simulink model "funcion_5"  (R2019a)
settings: Solver=VariableStepAuto  StartTime=0.0  StopTime=1  RelTol=1e-3
values from neighbouring files (symbols this model uses):
  a = -2.0000e-01    (= -0.2)    [programa_nodos.m]
  h = 1.0000e+00    (= 1)    [programa_nodos.m]
  hdis = hdis'    [programa_nodos.m]
  i = 1.0000e+00    (= 1)    [programa_nodos.m]
  j = 1.0000e+00    (= 1)    [programa_nodos.m]
  o = 1.0000e+00    (= 1)    [programa_nodos.m]
  s = 1.3156e+02    (= 131.56)    [programa_nodos.m]
  tm = 0.5    [programa_nodos.m]
  v = 1.2563e+00    (= 1.2563)    [programa_nodos.m]
  z0 = 0.5    [programa_nodos.m]
  z1 = 0.00000001    (= 1e-08)    [programa_nodos.m]
  z2 = 0.00000001    (= 1e-08)    [programa_nodos.m]
  z3 = 0.00000001    (= 1e-08)    [programa_nodos.m]
  z4 = 0.00000001    (= 1e-08)    [programa_nodos.m]
  z5 = 0.00000001    (= 1e-08)    [programa_nodos.m]
  z6 = 0.00000001    (= 1e-08)    [programa_nodos.m]
  z7 = 0.00000001    (= 1e-08)    [programa_nodos.m]
undefined symbols (not defined in the file or in its folder): A, A2, adis, B, B2, bdis, C, C2, cdis, g
libraries: simulink x1
settings Model: Creator=Alejoxbg  LastModifiedBy=Alejoxbg

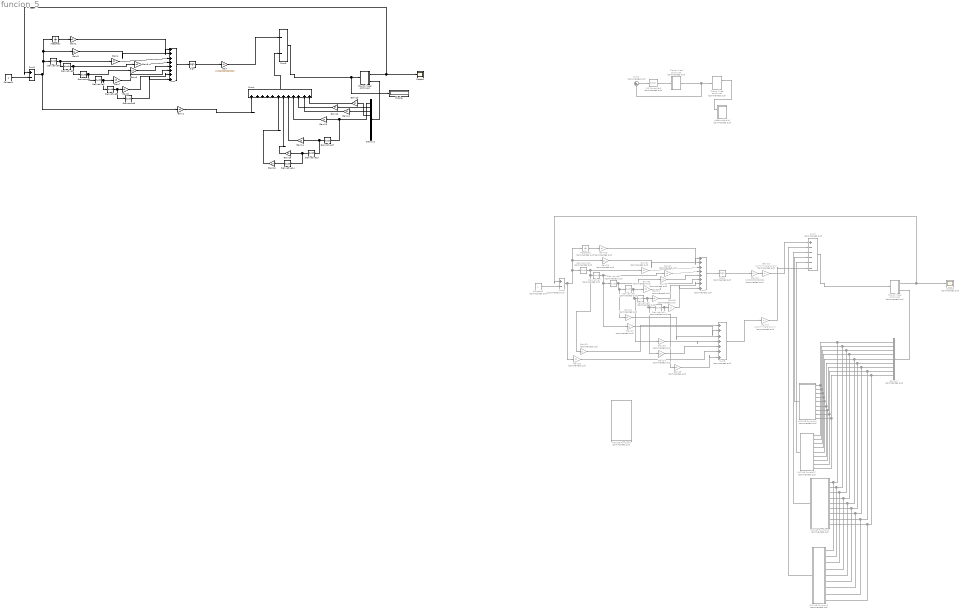
== system funcion_5 ==
  Constant : Constant
  Constant1 : Constant  Commented=on
  Demux1 : Demux  Commented=on  Outputs=9
  Demux2 : Demux  Outputs=9
  Derivative{1..6,13..14,17} (9 alike) : Derivative
  Derivative{7..12} (6 alike) : Derivative  Commented=on
  Display : Display
  Gain : Gain  Gain=0.0000000000001
  Gain1 : Gain  Gain=z0
  Gain10 : Gain  Gain=z1
  Gain11 : Gain  Gain=z2
  Gain12 : Gain  Gain=z3
  Gain13 : Gain  Gain=z4
  Gain14 : Gain  Gain=z5
  Gain15 : Gain  Gain=z6
  Gain16 : Gain  Gain=z7
  Gain18 : Gain  Commented=on  Gain=0.0000000000001
  Gain19 : Gain  Commented=on  Gain=1/(s*j*i*h*g*a*g*o*v)
  Gain2 : Gain  Gain=z0
  Gain20 : Gain  Commented=on  Gain=z1
  Gain21 : Gain  Commented=on  Gain=z2
  Gain22 : Gain  Commented=on  Gain=z3
  Gain23 : Gain  Commented=on  Gain=z4
  Gain24 : Gain  Commented=on  Gain=z5
  Gain25 : Gain  Commented=on  Gain=z6
  Gain26 : Gain  Commented=on  Gain=z0
  Gain27 : Gain  Commented=on  Gain=1/(s*j*i*h*g*a*g*o*v)
  Gain28 : Gain  Commented=on  Gain=z0
  Gain29 : Gain  Commented=on  Gain=z1
  Gain3 : Gain  Gain=z1
  Gain30 : Gain  Commented=on  Gain=z2
  Gain31 : Gain  Commented=on  Gain=z3
  Gain32 : Gain  Commented=on  Gain=z4
  Gain33 : Gain  Commented=on  Gain=z5
  Gain34 : Gain  Commented=on  Gain=z6
  Gain35 : Gain  Commented=on  Gain=z7
  Gain4 : Gain  Gain=z2
  Gain5 : Gain  Gain=z3
  Gain6 : Gain  Gain=z4
  Gain7 : Gain  Gain=z5
  Gain8 : Gain  Gain=z6
  Integrator : Integrator
  Integrator1 : Integrator  Commented=on
  MATLAB Function5 : MATLAB Function  Commented=on  TreatAsAtomicUnit=on
  MATLAB Function6 : MATLAB Function  Commented=on  TreatAsAtomicUnit=on
  MATLAB Function7 : MATLAB Function  Commented=on  TreatAsAtomicUnit=on
  MATLAB Function8 : MATLAB Function  Commented=on  TreatAsAtomicUnit=on
  MATLAB Function9 : MATLAB Function  Commented=on  TreatAsAtomicUnit=on
  PID Controller2 : simulink/Continuous/PID Controller  Commented=on  Controller=PID  Form=Parallel  TimeDomain=Continuous-time  SampleTime=-1  IntegratorMethod=Forward Euler  FilterMethod=Forward Euler  ControllerParametersSource=internal  P=12.1148539818802  I=1.25631014904339  D=27.6845650272969  UseFilter=on  N=4.3146205312046  TunerSelectOption=Transfer Function Based (PID Tuner App)  InitialConditionSource=internal  InitialConditionForIntegrator=0  InitialConditionForFilter=0  DifferentiatorICPrevScaledInput=0  ExternalReset=none  TrackingMode=off  Kt=1  LimitOutput=off  UpperSaturationLimit=inf  LowerSaturationLimit=-inf  LinearizeAsGain=on  AntiWindupMode=none  Kb=1  POutMin=[]  POutMax=[]  IOutMin=[]  IOutMax=[]  DOutMin=[]  DOutMax=[]  NOutMin=[]  NOutMax=[]  SumOutMin=[]  SumOutMax=[]  SaturationOutMin=[]  SaturationOutMax=[]  PParamMin=[]  PParamMax=[]  IParamMin=[]  IParamMax=[]  DParamMin=[]  DParamMax=[]  NParamMin=[]  NParamMax=[]  KbParamMin=[]  KbParamMax=[]  KtParamMin=[]  KtParamMax=[]  KbOutMin=[]  KbOutMax=[]  KtOutMin=[]  KtOutMax=[]  IntegratorOutMin=[]  IntegratorOutMax=[]  FilterOutMin=[]  FilterOutMax=[]  SumI1OutMin=[]  SumI1OutMax=[]  SumI2OutMin=[]  SumI2OutMax=[]  SumI3OutMin=[]  SumI3OutMax=[]  SumI4OutMin=[]  SumI4OutMax=[]  SumDOutMin=[]  SumDOutMax=[]  DifferentiatorOutMin=[]  DifferentiatorOutMax=[]  FilterDiffOutCoefMin=[]  FilterDiffOutCoefMax=[]  ReciprocalOutMin=[]  ReciprocalOutMax=[]  SumDenOutMin=[]  SumDenOutMax=[]  SumNumOutMin=[]  SumNumOutMax=[]  DivideOutMin=[]  DivideOutMax=[]  IntegratorContinuousStateAttributes=''  IntegratorStateMustResolveToSignalObject=off  IntegratorRTWStateStorageClass=Auto  FilterContinuousStateAttributes=''  FilterStateMustResolveToSignalObject=off  FilterRTWStateStorageClass=Auto  ParallelPVariant=InternalParameters  IdealPVariant=Disabled  IVariant=InternalParameters  DVariant=InternalParameters  IntegratorVariant=Continuous  SatVariant=Disabled  AWVariant=Passthrough  PCopyVariant=Disabled  TRVariant=Disabled  FdbkBlocksVariant=Forward  IdealPFdbkVariant=Disabled  SatFdbkVariant=Disabled  DerivativeFilterVariant=ContFilter  NVariant=InternalParameters  NCopyVariant=Disabled  FilterICVariant=InternalICsFilter  IntegratorICVariant=InternalICs  ExternalResetVariant=Disabled  TRSumVariant=Passthrough  SumFdbkVariant=Disabled  SumVariant=Sum_PID
  Planta lineal continua1 : Subsystem
  Planta lineal continua2 : Subsystem  Commented=on
  Planta lineal continua3 : Subsystem  Commented=on
  Planta lineal continua4 : Subsystem  Commented=on
  Scope1 : Scope
  Scope2 : Scope  Commented=on
  Sign : Signum  ZeroCross=off
  Sign1 : Signum  Commented=on  ZeroCross=off
  Sum : Sum  Inputs=|++++++++
  Sum1 : Sum  Commented=on  Inputs=|+-
  Sum2 : Sum  Inputs=|+-
  Sum3 : Sum  Inputs=|--
  Sum4 : Sum  Inputs=|++++++++++++
  Sum5 : Sum  Commented=on  Inputs=|++++++++
  Sum6 : Sum  Commented=on  Inputs=|+-
  Sum7 : Sum  Commented=on  Inputs=|+-----
  Sum8 : Sum  Commented=on  Inputs=|+++++++
  observadordis1 : Subsystem  Commented=on
  wires:
  Constant/1 -> Sum2/2
  Sum2/1 -> Gain1/1, Derivative6/1, Gain3/1, Integrator/1
  Integrator/1 -> Gain2/1
  Sum/1 -> Sign/1
  Sign/1 -> Gain/1
  Gain2/1 -> Sum/1
  Gain3/1 -> Sum/2
  Gain4/1 -> Sum/3
  Derivative6/1 -> Derivative1/1, Gain4/1
  Gain5/1 -> Sum/4
  Derivative1/1 -> Derivative4/1, Gain5/1
  Derivative4/1 -> Derivative2/1, Gain6/1
  Gain6/1 -> Sum/5
  Derivative2/1 -> Derivative3/1, Gain7/1
  Gain7/1 -> Sum/6
  Derivative3/1 -> Derivative5/1, Gain8/1
  Gain8/1 -> Sum/7
  Derivative5/1 -> Sum/8
  Gain/1 -> Sum3/1
  Sum3/1 -> Display/1, Planta lineal continua1/1(u)
  Sum1/1 -> PID Controller2/1
  Planta lineal continua3/1(y) -> Planta lineal continua4/1(u), Sum1/2
  ? -> Sum1/1
  PID Controller2/1 -> Planta lineal continua3/1(u)
  Planta lineal continua1/1(y) -> Sum2/1, Scope1/1
  Sum4/1 -> Sum3/2
  Gain23/1 -> Sum8/4
  Gain27/1 -> Sum7/6
  Demux1/8 -> MATLAB Function9/8(u8), MATLAB Function8/8(u8), MATLAB Function7/8(u8), MATLAB Function6/8(u8)
  Demux1/9 -> MATLAB Function9/9(u9), MATLAB Function8/9(u9), MATLAB Function7/9(u9), MATLAB Function6/9(u9)
  Gain33/1 -> Sum5/6
  Demux1/6 -> MATLAB Function9/6(u6), MATLAB Function8/6(u6), MATLAB Function7/6(u6), MATLAB Function6/6(u6)
  MATLAB Function6/1(y) -> Sum7/4
  MATLAB Function9/1(y) -> Sum7/2
  Demux1/2 -> MATLAB Function9/2(u2), MATLAB Function8/2(u2), MATLAB Function7/2(u2), MATLAB Function6/2(u2)
  Demux1/3 -> MATLAB Function9/3(u3), MATLAB Function8/3(u3), MATLAB Function7/3(u3), MATLAB Function6/3(u3)
  Gain29/1 -> Sum5/2
  Gain35/1 -> Sum5/8
  Sign1/1 -> Gain18/1
  Gain28/1 -> Sum5/1
  Gain34/1 -> Sum5/7
  Gain31/1 -> Sum5/4
  Constant1/1 -> Sum6/2
  Gain24/1 -> Sum8/5
  Derivative9/1 -> Gain24/1, Derivative11/1, Gain34/1
  Derivative10/1 -> Gain22/1, Derivative8/1, Gain32/1
  Demux1/4 -> MATLAB Function9/4(u4), MATLAB Function8/4(u4), MATLAB Function7/4(u4), MATLAB Function6/4(u4)
  Sum6/1 -> Gain26/1, Derivative12/1, Gain29/1, Integrator1/1
  Gain32/1 -> Sum5/5
  Planta lineal continua2/2(X) -> Demux1/1
  Gain25/1 -> Sum8/7
  Derivative8/1 -> Gain23/1, Derivative9/1, Gain33/1
  Planta lineal continua2/1(y) -> Sum6/1, Scope2/1
  Gain20/1 -> Sum8/1
  Gain21/1 -> Sum8/2
  Sum8/1 -> Gain27/1
  Demux1/5 -> MATLAB Function9/5(u5), MATLAB Function8/5(u5), MATLAB Function7/5(u5), MATLAB Function6/5(u5)
  Demux1/1 -> MATLAB Function9/1(u1), MATLAB Function8/1(u1), MATLAB Function7/1(u1), MATLAB Function6/1(u1)
  Demux1/7 -> MATLAB Function9/7(u7), MATLAB Function8/7(u7), MATLAB Function7/7(u7), MATLAB Function6/7(u7)
  Sum7/1 -> Planta lineal continua2/1(u)
  Derivative11/1 -> Gain25/1, Gain35/1
  Gain26/1 -> Sum8/6
  Gain30/1 -> Sum5/3
  Gain18/1 -> Gain19/1
  MATLAB Function7/1(y) -> Sum7/5
  Gain22/1 -> Sum8/3
  Derivative7/1 -> Gain21/1, Derivative10/1, Gain31/1
  MATLAB Function8/1(y) -> Sum7/3
  Gain19/1 -> Sum7/1
  Integrator1/1 -> Gain28/1
  Sum5/1 -> Sign1/1
  Derivative12/1 -> Gain20/1, Derivative7/1, Gain30/1
  Gain1/1 -> Sum4/1
  Planta lineal continua1/2(X) -> Demux2/1
  Demux2/4 -> Gain10/1
  Gain10/1 -> Sum4/12
  Demux2/3 -> Gain11/1
  Gain11/1 -> Sum4/11
  Demux2/2 -> Gain12/1
  Gain12/1 -> Sum4/10
  Gain13/1 -> Sum4/9
  Derivative17/1 -> Derivative13/1, Gain14/1
  Gain14/1 -> Sum4/8
  Gain15/1 -> Sum4/7
  Derivative14/1 -> Gain16/1
  Derivative13/1 -> Derivative14/1, Gain15/1
  Gain16/1 -> Sum4/6
  Planta lineal continua4/1(y) -> observadordis1/1(Y)
  ? -> observadordis1/2(U)
  Demux2/1 -> Derivative17/1, Gain13/1

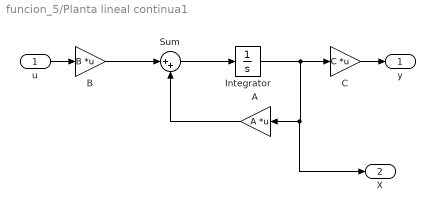
== system funcion_5/Planta lineal continua1 ==
  u : Inport
  A : Gain  Gain=A  Multiplication=Matrix(K*u) (u vector)
  B : Gain  Gain=B  Multiplication=Matrix(K*u) (u vector)
  C : Gain  Gain=C  Multiplication=Matrix(K*u) (u vector)
  Integrator : Integrator  InitialCondition=0.000001
  Sum : Sum  Inputs=|++
  y : Outport
  X : Outport  Port=2
  wires:
  C/1 -> y/1
  u/1 -> B/1
  Integrator/1 -> X/1, A/1, C/1
  A/1 -> Sum/2
  Sum/1 -> Integrator/1
  B/1 -> Sum/1

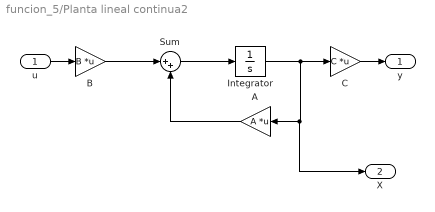
== system funcion_5/Planta lineal continua2 ==
  u : Inport
  A : Gain  Gain=A  Multiplication=Matrix(K*u) (u vector)
  B : Gain  Gain=B  Multiplication=Matrix(K*u) (u vector)
  C : Gain  Gain=C  Multiplication=Matrix(K*u) (u vector)
  Integrator : Integrator
  Sum : Sum  Inputs=|++
  y : Outport
  X : Outport  Port=2
  wires:
  C/1 -> y/1
  u/1 -> B/1
  Integrator/1 -> X/1, A/1, C/1
  A/1 -> Sum/2
  Sum/1 -> Integrator/1
  B/1 -> Sum/1

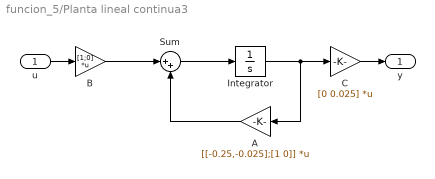
== system funcion_5/Planta lineal continua3 ==
  u : Inport
  A : Gain  Gain=[[-0.25,-0.025];[1 0]]  Multiplication=Matrix(K*u) (u vector)
  B : Gain  Gain=[1;0]  Multiplication=Matrix(K*u) (u vector)
  C : Gain  Gain=[0 0.025]  Multiplication=Matrix(K*u) (u vector)
  Integrator : Integrator
  Sum : Sum  Inputs=|++
  y : Outport
  wires:
  C/1 -> y/1
  u/1 -> B/1
  Integrator/1 -> A/1, C/1
  A/1 -> Sum/2
  Sum/1 -> Integrator/1
  B/1 -> Sum/1

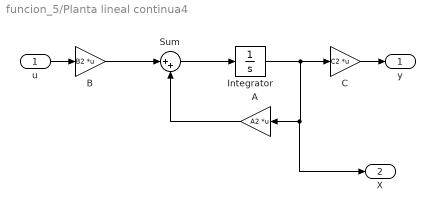
== system funcion_5/Planta lineal continua4 ==
  u : Inport
  A : Gain  Gain=A2  Multiplication=Matrix(K*u) (u vector)
  B : Gain  Gain=B2  Multiplication=Matrix(K*u) (u vector)
  C : Gain  Gain=C2  Multiplication=Matrix(K*u) (u vector)
  Integrator : Integrator
  Sum : Sum  Inputs=|++
  y : Outport
  X : Outport  Port=2
  wires:
  C/1 -> y/1
  u/1 -> B/1
  Integrator/1 -> X/1, A/1, C/1
  A/1 -> Sum/2
  Sum/1 -> Integrator/1
  B/1 -> Sum/1

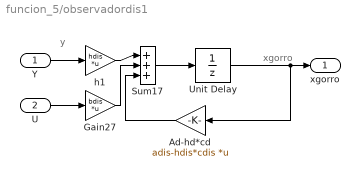
== system funcion_5/observadordis1 ==
  note: xgorro
  note: y
  Y : Inport
  U : Inport  Port=2
  Ad-hd*cd : Gain  Gain=adis-hdis*cdis  Multiplication=Matrix(K*u) (u vector)  SampleTime=tm
  Gain27 : Gain  Gain=bdis  Multiplication=Matrix(K*u) (u vector)  SampleTime=tm
  Sum17 : Sum  Inputs=|+++
  Unit Delay : UnitDelay  SampleTime=tm  HasFrameUpgradeWarning=on
  h1 : Gain  Gain=hdis  Multiplication=Matrix(K*u) (u vector)  SampleTime=tm
  xgorro : Outport
  wires:
  Sum17/1 -> Unit Delay/1
  h1/1 -> Sum17/1
  Unit Delay/1 -> Ad-hd*cd/1, xgorro/1
  Ad-hd*cd/1 -> Sum17/3
  Gain27/1 -> Sum17/2
  Y/1 -> h1/1
  U/1 -> Gain27/1

== matlab function funcion_5/MATLAB Function5 ==
  data: u1 input; y output; u2 input; u3 input; u4 input; u5 input; u6 input; u7 input; u8 input; u9 input
function y = fcn(u1,u2,u3,u4,u5,u6,u7,u8,u9)
  a=1.1520e-07
 b=-2.0000e-01
 c=-1.6000e-02  
 d=-6.4000e-04  
 e=-1.2800e-05  
 f=-1.0240e-07 
 g=2.5000e-02
 h=1.0000e+00
 i=1.0000e+00
 j=1.0000e+00
 k=1.0000e+00
 l=-2.5000e-01
 m=-3.3141e+00
 n=-4.3146e+00
 o=1.0000e+00
 p=1.0000e+00
 q=-2.9862e+00
 r=-4.3146e+00
 s=-3.1408e-02
 t=1.3156e+02
 u=1.1945e+02
 v=1.2563e+00
y = s*j*i*h*g*a*a*(a*u1+b*u2+c*u3+d*u4+e*u5+g*u7)+s*j*i*h*g*a*(b*g*u1+c*h*u2+d*i*u3+e*j*u4+g*o*u6)+s*j*i*h*g*a*(d*h*g*u1+d*h*u2+d*i*u3)+s*j*i*h*g*a*g*o*(k*u6+l*u7+m*u8+n*u9)+s*j*i*h*g*a*g*o*v*u;

== matlab function funcion_5/MATLAB Function6 ==
  data: u1 input; y output; u2 input; u3 input; u4 input; u5 input; u6 input; u7 input; u8 input; u9 input
function y = fcn(u1,u2,u3,u4,u5,u6,u7,u8,u9)
a=1.1520e-07
 b=-2.0000e-01
 c=-1.6000e-02  
 d=-6.4000e-04  
 e=-1.2800e-05  
 f=-1.0240e-07 
 g=2.5000e-02
 h=1.0000e+00
 i=1.0000e+00
 j=1.0000e+00
 k=1.0000e+00
 l=-2.5000e-01
 m=-3.3141e+00
 n=-4.3146e+00
 o=1.0000e+00
 p=1.0000e+00
 q=-2.9862e+00
 r=-4.3146e+00
 s=-3.1408e-02
 t=1.3156e+02
 u=1.1945e+02
 v=1.2563e+00
y = a/(g*o*v)*(a*u1+b*u2+c*u3+d*u4+e*u5+g*u6);

== matlab function funcion_5/MATLAB Function7 ==
  data: u1 input; y output; u2 input; u3 input; u4 input; u5 input; u6 input; u7 input; u8 input; u9 input
function y = fcn(u1,u2,u3,u4,u5,u6,u7,u8,u9)
a=1.1520e-07
 b=-2.0000e-01
 c=-1.6000e-02  
 d=-6.4000e-04  
 e=-1.2800e-05  
 f=-1.0240e-07 
 g=2.5000e-02
 h=1.0000e+00
 i=1.0000e+00
 j=1.0000e+00
 k=1.0000e+00
 l=-2.5000e-01
 m=-3.3141e+00
 n=-4.3146e+00
 o=1.0000e+00
 p=1.0000e+00
 q=-2.9862e+00
 r=-4.3146e+00
 s=-3.1408e-02
 t=1.3156e+02
 u=1.1945e+02
 v=1.2563e+00
y = 1/(g*o*v)*(b*g*u1+c*h*u2+d*i*u3+e*j*u4+g*o*u6);

== matlab function funcion_5/MATLAB Function8 ==
  data: u1 input; y output; u2 input; u3 input; u4 input; u5 input; u6 input; u7 input; u8 input; u9 input
function y= fcn(u1,u2,u3,u4,u5,u6,u7,u8,u9)
a=1.1520e-07
 b=-2.0000e-01
 c=-1.6000e-02  
 d=-6.4000e-04  
 e=-1.2800e-05  
 f=-1.0240e-07 
 g=2.5000e-02
 h=1.0000e+00
 i=1.0000e+00
 j=1.0000e+00
 k=1.0000e+00
 l=-2.5000e-01
 m=-3.3141e+00
 n=-4.3146e+00
 o=1.0000e+00
 p=1.0000e+00
 q=-2.9862e+00
 r=-4.3146e+00
 s=-3.1408e-02
 t=1.3156e+02
 u=1.1945e+02
 v=1.2563e+00
y = 1/(g*o*v)*(d*h*g*u1+c*h*u2+d*i*u3);

== matlab function funcion_5/MATLAB Function9 ==
  data: u1 input; y output; u2 input; u3 input; u4 input; u5 input; u6 input; u7 input; u8 input; u9 input
function y = fcn(u1,u2,u3,u4,u5,u6,u7,u8,u9)
a=1.1520e-07
 b=-2.0000e-01
 c=-1.6000e-02  
 d=-6.4000e-04  
 e=-1.2800e-05  
 f=-1.0240e-07 
 g=2.5000e-02
 h=1.0000e+00
 i=1.0000e+00
 j=1.0000e+00
 k=1.0000e+00
 l=-2.5000e-01
 m=-3.3141e+00
 n=-4.3146e+00
 o=1.0000e+00
 p=1.0000e+00
 q=-2.9862e+00
 r=-4.3146e+00
 s=-3.1408e-02
 t=1.3156e+02
 u=1.1945e+02
 v=1.2563e+00
y = 1/(v)*(k*u6+l*u7+m*u8+n*u9);
